simulink model "State_Flow_D"  (R2017a)
settings: Solver=FixedStepDiscrete  StartTime=0.0  StopTime=inf  FixedStep=0.001  RelTol=1e-3  EnableMultiTasking=on
libraries: xpcethercatlib x35, simulink x11, commutil2 x2
(part 3 of 3)

== matlab function State_Flow_D/Movimento/MATLAB Jin ==
  data: x input; y input; theta1 input; x_p output; theta2 input; theta1_p input; theta2_p input; y_p output
function [x_p, y_p] = fcn(x, y, theta1, theta2, theta1_p, theta2_p)

d = 0.09; 
l = 0.25;

N21 = -l*sin(theta1)*(x+d-l*cos(theta1)) + l*cos(theta1)*(y-l*sin(theta1));

N22 = -l*cos(theta2)*(y-l*sin(theta2))*(x+d-l*cos(theta1))/(x-d-l*cos(theta2)) + l*sin(theta2)*(x+d-l*cos(theta1));

D2 = y-l*sin(theta1) - (y-l*sin(theta2))*(x+d-l*cos(theta1))/(x-d-l*cos(theta2));

J21 = N21/D2;

J22 = N22/D2;

J11 = -(y-l*sin(theta2))/(x-d-l*cos(theta2))*(J21);

J12 = -(y-l*sin(theta2))/(x-d-l*cos(theta2))*(J22) -l*sin(theta2) + (y-l*sin(theta2))/(x-d-l*cos(theta2))*(l*cos(theta2));

x_p = J11*theta1_p + J12*theta2_p;
y_p = J21*theta1_p + J22*theta2_p;

== matlab function State_Flow_D/Movimento/Leggi di moto/Cerchio ==
  data: xc output; t input; yc output; T input; r input; xc_p output; yc_p output; xc_pp output; yc_pp output
function [xc, yc, xc_p, yc_p, xc_pp, yc_pp] = fcn(t, T, r)
xv = 0.4;
xj = 0.1;
x = t/T;
Ca = 1/((1-xv)*(xv-xj));
if ( x >= 0 && x < xj)            %acc crescente positiva
    f = Ca/xj*x;
    F = (1/2)*Ca/xj*x^2;
    G = (1/6)*Ca/xj*x^3;
    J = Ca/xj;

  elseif (x >= xj && x < (xv-xj))   %acc costante positiva
    f = Ca;
    F = Ca*x - (1/2)*Ca*xj;
    G = (1/2)*Ca*x^2 - (1/2)*Ca*xj*x + (1/6)*Ca*xj^2;
    J = 0;

  elseif( x>= (xv-xj) && x < xv)    %acc decrescente positiva
    f = -Ca/xj*x + Ca*xv/xj;
    F = -(1/2)*Ca/xj*x^2 + Ca/xj*xv*x - Ca*(xj + (1/2)/xj*xv^2 - xv);
    G = -(1/6)*Ca/xj*x^3 + (1/2)*Ca/xj*xv*x^2 - Ca*(xj + (1/2)/xj*xv^2 - xv)*x ...
        - (1/2)*Ca*xv^2  + (1/6)*Ca/xj*xv^3 + (1/2)*Ca*xv*xj;
    J = -Ca/xj;

  elseif( x>= xv && x < (1-xv))     %acc costante nulla
    f = 0;
    F = Ca*(xv - xj);
    G = Ca*(xv - xj)*x - (1/2)*Ca*xv^2 + (1/2)*Ca*xv*xj;
    J = 0;
    
  elseif( x>= (1-xv) && x < (1-xv+xj))   %acc decrescente negativa
    f = -Ca/xj*x + Ca/xj*(1-xv);
    F = -(1/2)*Ca/xj*x^2 + Ca/xj*(1-xv)*x + Ca*(xv-xj) - (1/2)*Ca/xj*(1-xv)^2;
    G = -(1/6)*Ca/xj*x^3 + (1/2)*Ca/xj*(1-xv)*x^2 + Ca*(xv-xj)*x - (1/2)*Ca/xj*(1-xv)^2*x ...
        - (1/2)*Ca*xv^2 + (1/2)*Ca*xv*xj + (1/6)*Ca/xj*(1-xv)^3;
    J = -Ca/xj;
    
  elseif( x>= (1-xv+xj) && x < (1-xj))   %acc costante negativa
    f = -Ca; 
    F = -Ca*x + Ca - (1/2)*Ca*xj;
    G = -(1/2)*Ca*x^2 + Ca*x - (1/2)*Ca*xj*x + 1 - Ca*(-(1/2)*xj + (1/6)*xj^2 + (1/2));
    J = 0;
    
  elseif( x>= (1-xj) && x <= 1)          %acc crescente negativa
    f = Ca/xj*(x-1);
    F = (1/2)*Ca/xj*x^2 - Ca/xj*x +(1/2)*Ca/xj;
    G = (1/6)*Ca/xj*x^3 - (1/2)*Ca/xj*x^2 +(1/2)*Ca/xj*x + 1 - (1/6)*Ca/xj;
    J = Ca/xj;
    
  else                                   %acc costante nulla
    f = 0;
    F = 0;
    G = 1;
    J = 0;
end
  
 alfa = G*2*pi;
 alfa_p = F*2*pi/T;
 alfa_pp = f*2*pi/(T^2);
 xc = r*cos(pi/2-alfa);
 yc = r*sin(pi/2-alfa) - r;
 xc_p = r*sin(pi/2-alfa)*alfa_p;
 yc_p = -r*cos(pi/2-alfa)*alfa_p;
 xc_pp = -r*cos(pi/2-alfa)*alfa_p^2 + r*sin(pi/2-alfa)*alfa_pp;
 yc_pp = -r*sin(pi/2-alfa)*alfa_p^2- r*cos(pi/2-alfa)*alfa_pp;

== matlab function State_Flow_D/Movimento/Leggi di moto/Quadrato ==
  data: xq output; yq output; t input; T input; h input; xq_p output; yq_p output; xq_pp output; yq_pp output
function [xq, yq, xq_p, yq_p, xq_pp, yq_pp] = fcn(t, T, h)
xv = 0.4;
xj = 0.1;
x1 = t/(0.5*T/4);
x2 = (t-0.5*T/4)/(T/4);
x3 = (t-1.5*T/4)/(T/4);
x4 = (t-2.5*T/4)/(T/4);
x5 = (t-3.5*T/4)/(0.5*T/4);
Ca = 1/((1-xv)*(xv-xj));
% Ca = 1/(xv*(1-xv));
% Cv = 1/(1-xv);


if t > 0 && t <= 0.5*T/4
  
  if ( x1 >= 0 && x1 < xj)            %acc crescente positiva
    f = Ca/xj*x1;
    F = (1/2)*Ca/xj*x1^2;
    G = (1/6)*Ca/xj*x1^3;
    J = Ca/xj;

  elseif (x1 >= xj && x1 < (xv-xj))   %acc costante positiva
    f = Ca;
    F = Ca*x1 - (1/2)*Ca*xj;
    G = (1/2)*Ca*x1^2 - (1/2)*Ca*xj*x1 + (1/6)*Ca*xj^2;
    J = 0;

  elseif( x1>= (xv-xj) && x1 < xv)    %acc decrescente positiva
    f = -Ca/xj*x1 + Ca*xv/xj;
    F = -(1/2)*Ca/xj*x1^2 + Ca/xj*xv*x1 - Ca*(xj + (1/2)/xj*xv^2 - xv);
    G = -(1/6)*Ca/xj*x1^3 + (1/2)*Ca/xj*xv*x1^2 - Ca*(xj + (1/2)/xj*xv^2 - xv)*x1 ...
        - (1/2)*Ca*xv^2  + (1/6)*Ca/xj*xv^3 + (1/2)*Ca*xv*xj;
    J = -Ca/xj;

  elseif( x1>= xv && x1 < (1-xv))     %acc costante nulla
    f = 0;
    F = Ca*(xv - xj);
    G = Ca*(xv - xj)*x1 - (1/2)*Ca*xv^2 + (1/2)*Ca*xv*xj;
    J = 0;
    
  elseif( x1>= (1-xv) && x1 < (1-xv+xj))   %acc decrescente negativa
    f = -Ca/xj*x1 + Ca/xj*(1-xv);
    F = -(1/2)*Ca/xj*x1^2 + Ca/xj*(1-xv)*x1 + Ca*(xv-xj) - (1/2)*Ca/xj*(1-xv)^2;
    G = -(1/6)*Ca/xj*x1^3 + (1/2)*Ca/xj*(1-xv)*x1^2 + Ca*(xv-xj)*x1 - (1/2)*Ca/xj*(1-xv)^2*x1 ...
        - (1/2)*Ca*xv^2 + (1/2)*Ca*xv*xj + (1/6)*Ca/xj*(1-xv)^3;
    J = -Ca/xj;
    
  elseif( x1>= (1-xv+xj) && x1 < (1-xj))   %acc costante negativa
    f = -Ca; 
    F = -Ca*x1 + Ca - (1/2)*Ca*xj;
    G = -(1/2)*Ca*x1^2 + Ca*x1 - (1/2)*Ca*xj*x1 + 1 - Ca*(-(1/2)*xj + (1/6)*xj^2 + (1/2));
    J = 0;
    
  elseif( x1>= (1-xj) && x1 <= 1)          %acc crescente negativa
    f = Ca/xj*(x1-1);
    F = (1/2)*Ca/xj*x1^2 - Ca/xj*x1 +(1/2)*Ca/xj;
    G = (1/6)*Ca/xj*x1^3 - (1/2)*Ca/xj*x1^2 +(1/2)*Ca/xj*x1 + 1 - (1/6)*Ca/xj;
    J = Ca/xj;
    
  else                                   %acc costante nulla
    f = 0;
    F = 0;
    G = 1;
    J = 0;
  end
    xq = G*h/2;
    xq_p = F*(h/2)/(T/4);
    yq = 0;
    yq_p = 0; 
    xq_pp = f*(h/2)/((T/4)^2);
    yq_pp = 0;

elseif t > 0.5*T/4 && t <= 1.5*T/4
    Ca = 1/((1-xv)*(xv-xj));
% Cj = Ca/xj;
  
  if ( x2 >= 0 && x2 < xj)            %acc crescente positiva
    f = Ca/xj*x2;
    F = (1/2)*Ca/xj*x2^2;
    G = (1/6)*Ca/xj*x2^3;
    J = Ca/xj;

  elseif (x2 >= xj && x2 < (xv-xj))   %acc costante positiva
    f = Ca;
    F = Ca*x2 - (1/2)*Ca*xj;
    G = (1/2)*Ca*x2^2 - (1/2)*Ca*xj*x2 + (1/6)*Ca*xj^2;
    J = 0;

  elseif( x2>= (xv-xj) && x2 < xv)    %acc decrescente positiva
    f = -Ca/xj*x2 + Ca*xv/xj;
    F = -(1/2)*Ca/xj*x2^2 + Ca/xj*xv*x2 - Ca*(xj + (1/2)/xj*xv^2 - xv);
    G = -(1/6)*Ca/xj*x2^3 + (1/2)*Ca/xj*xv*x2^2 - Ca*(xj + (1/2)/xj*xv^2 - xv)*x2 ...
        - (1/2)*Ca*xv^2  + (1/6)*Ca/xj*xv^3 + (1/2)*Ca*xv*xj;
    J = -Ca/xj;

  elseif( x2>= xv && x2 < (1-xv))     %acc costante nulla
    f = 0;
    F = Ca*(xv - xj);
    G = Ca*(xv - xj)*x2 - (1/2)*Ca*xv^2 + (1/2)*Ca*xv*xj;
    J = 0;
    
  elseif( x2>= (1-xv) && x2 < (1-xv+xj))   %acc decrescente negativa
    f = -Ca/xj*x2 + Ca/xj*(1-xv);
    F = -(1/2)*Ca/xj*x2^2 + Ca/xj*(1-xv)*x2 + Ca*(xv-xj) - (1/2)*Ca/xj*(1-xv)^2;
    G = -(1/6)*Ca/xj*x2^3 + (1/2)*Ca/xj*(1-xv)*x2^2 + Ca*(xv-xj)*x2 - (1/2)*Ca/xj*(1-xv)^2*x2 ...
        - (1/2)*Ca*xv^2 + (1/2)*Ca*xv*xj + (1/6)*Ca/xj*(1-xv)^3;
    J = -Ca/xj;
    
  elseif( x2>= (1-xv+xj) && x2 < (1-xj))   %acc costante negativa
    f = -Ca; 
    F = -Ca*x2 + Ca - (1/2)*Ca*xj;
    G = -(1/2)*Ca*x2^2 + Ca*x2 - (1/2)*Ca*xj*x2 + 1 - Ca*(-(1/2)*xj + (1/6)*xj^2 + (1/2));
    J = 0;
    
  elseif( x2>= (1-xj) && x2 <= 1)          %acc crescente negativa
    f = Ca/xj*(x2-1);
    F = (1/2)*Ca/xj*x2^2 - Ca/xj*x2 +(1/2)*Ca/xj;
    G = (1/6)*Ca/xj*x2^3 - (1/2)*Ca/xj*x2^2 +(1/2)*Ca/xj*x2 + 1 - (1/6)*Ca/xj;
    J = Ca/xj;
    
  else                                   %acc costante nulla
    f = 0;
    F = 0;
    G = 1;
    J = 0;
  end
    xq = h/2;
    xq_p = 0;
    yq = -G*h; 
    yq_p = -F*h/(T/4); 
    xq_pp = 0;
    yq_pp = -f*(h/2)/((T/4)^2);

elseif t > 1.5*T/4 && t <= 2.5*T/4
     Ca = 1/((1-xv)*(xv-xj));
% Cj = Ca/xj;
  
  if ( x3 >= 0 && x3 < xj)            %acc crescente positiva
    f = Ca/xj*x3;
    F = (1/2)*Ca/xj*x3^2;
    G = (1/6)*Ca/xj*x3^3;
    J = Ca/xj;

  elseif (x3 >= xj && x3 < (xv-xj))   %acc costante positiva
    f = Ca;
    F = Ca*x3 - (1/2)*Ca*xj;
    G = (1/2)*Ca*x3^2 - (1/2)*Ca*xj*x3 + (1/6)*Ca*xj^2;
    J = 0;

  elseif( x3>= (xv-xj) && x3 < xv)    %acc decrescente positiva
    f = -Ca/xj*x3 + Ca*xv/xj;
    F = -(1/2)*Ca/xj*x3^2 + Ca/xj*xv*x3 - Ca*(xj + (1/2)/xj*xv^2 - xv);
    G = -(1/6)*Ca/xj*x3^3 + (1/2)*Ca/xj*xv*x3^2 - Ca*(xj + (1/2)/xj*xv^2 - xv)*x3 ...
        - (1/2)*Ca*xv^2  + (1/6)*Ca/xj*xv^3 + (1/2)*Ca*xv*xj;
    J = -Ca/xj;

  elseif( x3>= xv && x3 < (1-xv))     %acc costante nulla
    f = 0;
    F = Ca*(xv - xj);
    G = Ca*(xv - xj)*x3 - (1/2)*Ca*xv^2 + (1/2)*Ca*xv*xj;
    J = 0;
    
  elseif( x3>= (1-xv) && x3 < (1-xv+xj))   %acc decrescente negativa
    f = -Ca/xj*x3 + Ca/xj*(1-xv);
    F = -(1/2)*Ca/xj*x3^2 + Ca/xj*(1-xv)*x3 + Ca*(xv-xj) - (1/2)*Ca/xj*(1-xv)^2;
    G = -(1/6)*Ca/xj*x3^3 + (1/2)*Ca/xj*(1-xv)*x3^2 + Ca*(xv-xj)*x3 - (1/2)*Ca/xj*(1-xv)^2*x3 ...
        - (1/2)*Ca*xv^2 + (1/2)*Ca*xv*xj + (1/6)*Ca/xj*(1-xv)^3;
    J = -Ca/xj;
    
  elseif( x3>= (1-xv+xj) && x3 < (1-xj))   %acc costante negativa
    f = -Ca; 
    F = -Ca*x3 + Ca - (1/2)*Ca*xj;
    G = -(1/2)*Ca*x3^2 + Ca*x3 - (1/2)*Ca*xj*x3 + 1 - Ca*(-(1/2)*xj + (1/6)*xj^2 + (1/2));
    J = 0;
    
  elseif( x3>= (1-xj) && x3 <= 1)          %acc crescente negativa
    f = Ca/xj*(x3-1);
    F = (1/2)*Ca/xj*x3^2 - Ca/xj*x3 +(1/2)*Ca/xj;
    G = (1/6)*Ca/xj*x3^3 - (1/2)*Ca/xj*x3^2 +(1/2)*Ca/xj*x3 + 1 - (1/6)*Ca/xj;
    J = Ca/xj;
    
  else                                   %acc costante nulla
    f = 0;
    F = 0;
    G = 1;
    J = 0;
  end
    xq = h/2-G*h;
    xq_p = -F*h/(T/4);
    yq = -h; 
    yq_p = 0; 
    xq_pp = -f*(h/2)/((T/4)^2);
    yq_pp = 0;
 
elseif t > 2.5*T/4 && t <= 3.5*T/4
   Ca = 1/((1-xv)*(xv-xj));
% Cj = Ca/xj;
  
  if ( x4 >= 0 && x4 < xj)            %acc crescente positiva
    f = Ca/xj*x4;
    F = (1/2)*Ca/xj*x4^2;
    G = (1/6)*Ca/xj*x4^3;
    J = Ca/xj;

  elseif (x4 >= xj && x4 < (xv-xj))   %acc costante positiva
    f = Ca;
    F = Ca*x4 - (1/2)*Ca*xj;
    G = (1/2)*Ca*x4^2 - (1/2)*Ca*xj*x4 + (1/6)*Ca*xj^2;
    J = 0;

  elseif( x4>= (xv-xj) && x4 < xv)    %acc decrescente positiva
    f = -Ca/xj*x4 + Ca*xv/xj;
    F = -(1/2)*Ca/xj*x4^2 + Ca/xj*xv*x4 - Ca*(xj + (1/2)/xj*xv^2 - xv);
    G = -(1/6)*Ca/xj*x4^3 + (1/2)*Ca/xj*xv*x4^2 - Ca*(xj + (1/2)/xj*xv^2 - xv)*x4 ...
        - (1/2)*Ca*xv^2  + (1/6)*Ca/xj*xv^3 + (1/2)*Ca*xv*xj;
    J = -Ca/xj;

  elseif( x4>= xv && x4 < (1-xv))     %acc costante nulla
    f = 0;
    F = Ca*(xv - xj);
    G = Ca*(xv - xj)*x4 - (1/2)*Ca*xv^2 + (1/2)*Ca*xv*xj;
    J = 0;
    
  elseif( x4>= (1-xv) && x4 < (1-xv+xj))   %acc decrescente negativa
    f = -Ca/xj*x4 + Ca/xj*(1-xv);
    F = -(1/2)*Ca/xj*x4^2 + Ca/xj*(1-xv)*x4 + Ca*(xv-xj) - (1/2)*Ca/xj*(1-xv)^2;
    G = -(1/6)*Ca/xj*x4^3 + (1/2)*Ca/xj*(1-xv)*x4^2 + Ca*(xv-xj)*x4 - (1/2)*Ca/xj*(1-xv)^2*x4 ...
        - (1/2)*Ca*xv^2 + (1/2)*Ca*xv*xj + (1/6)*Ca/xj*(1-xv)^3;
    J = -Ca/xj;
    
  elseif( x4>= (1-xv+xj) && x4 < (1-xj))   %acc costante negativa
    f = -Ca; 
    F = -Ca*x4 + Ca - (1/2)*Ca*xj;
    G = -(1/2)*Ca*x4^2 + Ca*x4 - (1/2)*Ca*xj*x4 + 1 - Ca*(-(1/2)*xj + (1/6)*xj^2 + (1/2));
    J = 0;
    
  elseif( x4>= (1-xj) && x4 <= 1)          %acc crescente negativa
    f = Ca/xj*(x4-1);
    F = (1/2)*Ca/xj*x4^2 - Ca/xj*x4 +(1/2)*Ca/xj;
    G = (1/6)*Ca/xj*x4^3 - (1/2)*Ca/xj*x4^2 +(1/2)*Ca/xj*x4 + 1 - (1/6)*Ca/xj;
    J = Ca/xj;
    
  else                                   %acc costante nulla
    f = 0;
    F = 0;
    G = 1;
    J = 0;
  end
    xq = -h/2;
    xq_p = 0;
    yq = -h + G*h;
    yq_p = F*h/(T/4); 
    xq_pp = 0;
    yq_pp = f*(h/2)/((T/4)^2);

elseif t > 3.5*T/4 && t <= 4*T/4
   Ca = 1/((1-xv)*(xv-xj));
% Cj = Ca/xj;
  
  if ( x5 >= 0 && x5 < xj)            %acc crescente positiva
    f = Ca/xj*x5;
    F = (1/2)*Ca/xj*x5^2;
    G = (1/6)*Ca/xj*x5^3;
    J = Ca/xj;

  elseif (x5 >= xj && x5 < (xv-xj))   %acc costante positiva
    f = Ca;
    F = Ca*x5 - (1/2)*Ca*xj;
    G = (1/2)*Ca*x5^2 - (1/2)*Ca*xj*x5 + (1/6)*Ca*xj^2;
    J = 0;

  elseif( x5>= (xv-xj) && x5 < xv)    %acc decrescente positiva
    f = -Ca/xj*x5 + Ca*xv/xj;
    F = -(1/2)*Ca/xj*x5^2 + Ca/xj*xv*x5 - Ca*(xj + (1/2)/xj*xv^2 - xv);
    G = -(1/6)*Ca/xj*x5^3 + (1/2)*Ca/xj*xv*x5^2 - Ca*(xj + (1/2)/xj*xv^2 - xv)*x5 ...
        - (1/2)*Ca*xv^2  + (1/6)*Ca/xj*xv^3 + (1/2)*Ca*xv*xj;
    J = -Ca/xj;

  elseif( x5>= xv && x5 < (1-xv))     %acc costante nulla
    f = 0;
    F = Ca*(xv - xj);
    G = Ca*(xv - xj)*x5 - (1/2)*Ca*xv^2 + (1/2)*Ca*xv*xj;
    J = 0;
    
  elseif( x5>= (1-xv) && x5 < (1-xv+xj))   %acc decrescente negativa
    f = -Ca/xj*x5 + Ca/xj*(1-xv);
    F = -(1/2)*Ca/xj*x5^2 + Ca/xj*(1-xv)*x5 + Ca*(xv-xj) - (1/2)*Ca/xj*(1-xv)^2;
    G = -(1/6)*Ca/xj*x5^3 + (1/2)*Ca/xj*(1-xv)*x5^2 + Ca*(xv-xj)*x5 - (1/2)*Ca/xj*(1-xv)^2*x5 ...
        - (1/2)*Ca*xv^2 + (1/2)*Ca*xv*xj + (1/6)*Ca/xj*(1-xv)^3;
    J = -Ca/xj;
    
  elseif( x5>= (1-xv+xj) && x5 < (1-xj))   %acc costante negativa
    f = -Ca; 
    F = -Ca*x5 + Ca - (1/2)*Ca*xj;
    G = -(1/2)*Ca*x5^2 + Ca*x5 - (1/2)*Ca*xj*x5 + 1 - Ca*(-(1/2)*xj + (1/6)*xj^2 + (1/2));
    J = 0;
    
  elseif( x5>= (1-xj) && x5 <= 1)          %acc crescente negativa
    f = Ca/xj*(x5-1);
    F = (1/2)*Ca/xj*x5^2 - Ca/xj*x5 +(1/2)*Ca/xj;
    G = (1/6)*Ca/xj*x5^3 - (1/2)*Ca/xj*x5^2 +(1/2)*Ca/xj*x5 + 1 - (1/6)*Ca/xj;
    J = Ca/xj;
    
  else                                   %acc costante nulla
    f = 0;
    F = 0;
    G = 1;
    J = 0;
  end
    xq = -h/2 + G*h/2;
    xq_p = F*h/2/(T/4);
    yq = 0
    yq_p = 0; 
    xq_pp = f*(h/2)/((T/4)^2);
    yq_pp = 0;
else
xq = 0;
yq = 0;
xq_p = 0;
yq_p = 0; 
xq_pp = 0;
yq_pp = 0;
end

== matlab function State_Flow_D/Movimento/Leggi di moto/g ==
  data: x output; y output; x_p output; t input; l input; T input; y_p output; x_pp output; y_pp output
function [x, y, x_p,y_p, x_pp, y_pp] = fcn(t, l, T)
 Tt = T/32;
 t1 = (t-0*Tt/2)/(Tt/2);
 t2 = (t-1*Tt/2)/Tt;
 t3 = (t-3*Tt/2)/(Tt/2);
 t4 = (t-4*Tt/2)/(Tt/2);
 t5 = (t-5*Tt/2)/Tt;
 t6 = (t-7*Tt/2)/Tt;
 t7 = (t-9*Tt/2)/Tt;
 t8 = (t-11*Tt/2)/(Tt/2);
 t9 = (t-12*Tt/2)/(Tt/2);
 t10 = (t-13*Tt/2)/Tt;
 t11 = (t-15*Tt/2)/(Tt/2);
 t12 = (t-16*Tt/2)/(Tt/2);
 t13 = (t-17*Tt/2)/Tt;
 t14 = (t-19*Tt/2)/(Tt/2);
 t15 = (t-20*Tt/2)/(Tt/2);
 t16 = (t-21*Tt/2)/Tt;
 t17 = (t-23*Tt/2)/Tt;
 t18 = (t-25*Tt/2)/Tt;
 t19 = (t-27*Tt/2)/(Tt/2);
 t20 = (t-28*Tt/2)/(Tt/2);
 t21 = (t-29*Tt/2)/Tt;
 t22 = (t-31*Tt/2)/(Tt/2);
 t23 = (t-32*Tt/2)/(Tt/2);
 t24 = (t-33*Tt/2)/Tt;
 t25 = (t-35*Tt/2)/(Tt/2);
 t26 = (t-36*Tt/2)/(Tt/2);
 t27 = (t-37*Tt/2)/Tt;
 t28 = (t-39*Tt/2)/Tt;
 t29 = (t-41*Tt/2)/Tt;
 t30 = (t-43*Tt/2)/(Tt/2);
 t31 = (t-44*Tt/2)/(Tt/2);
 t32 = (t-45*Tt/2)/Tt;
 t33 = (t-47*Tt/2)/(Tt/2);
 t34 = (t-48*Tt/2)/(Tt/2);
 t35 = (t-49*Tt/2)/Tt;
 t36 = (t-51*Tt/2)/(Tt/2);
 t37 = (t-52*Tt/2)/(Tt/2);
 t38 = (t-53*Tt/2)/Tt;
 t39 = (t-55*Tt/2)/Tt;
 t40 = (t-57*Tt/2)/Tt;
 t41 = (t-59*Tt/2)/(Tt/2);
 t42 = (t-60*Tt/2)/(Tt/2);
 t43 = (t-61*Tt/2)/Tt;
 t44 = (t-63*Tt/2)/(Tt/2);
 
 if t > 0 && t <= Tt/2 % 1
     [G, F, f] = ldm7t(t1);
     x = 0;
     x_p = 0;
     y = -G*l;
     y_p = -F*l/(Tt/2);
     x_pp = 0;
     y_pp = -f*l/((Tt/2)^2);
     
 elseif t > Tt/2 && t <= 3*Tt/2 % 2
     [G, F, f] = ldm7t(t2);
     x = G*3*l;
     x_p = F*3*l/Tt;
     y = -l;
     y_p = 0;
     x_pp = f*l/((Tt)^2);
     y_pp = 0;
     
 elseif t > 3*Tt/2 && t <= 4*Tt/2 % 3
     [G, F, f] = ldm7t(t3);
     x = 3*l;
     x_p = 0;
     y = -l + G*l;
     y_p = F*l/(Tt/2);
     x_pp = 0;
     y_pp = f*l/((Tt/2)^2);
     
  elseif t > 4*Tt/2 && t <= 5*Tt/2 % 4
     [G, F, f] = ldm7t(t4);
     x = 3*l - G*l;
     x_p = -F*l/(Tt/2);
     y = 0;
     y_p = 0;
     x_pp = -f*l/((Tt/2)^2);
     y_pp = 0;
     
  elseif t > 5*Tt/2 && t <= 7*Tt/2 % 5
     [G, F, f] = ldm7t(t5);
     x = 2*l;
     x_p = 0;
     y = -G*3*l;
     y_p = -F*3*l/Tt;
     x_pp = 0;
     y_pp = -f*l/((Tt)^2);
     
  elseif t > 7*Tt/2 && t <= 9*Tt/2 % 6
     [G, F, f] = ldm7t(t6);
     x = 2*l + G*3*l;
     x_p = F*3*l/Tt;
     y = -3*l;
     y_p = 0;
     x_pp = f*l/((Tt)^2);
     y_pp = 0;
     
  elseif t > 9*Tt/2 && t <= 11*Tt/2 % 7
     [G, F, f] = ldm7t(t7);
     x = 5*l;
     x_p = 0;
     y = -3*l + G*3*l;
     y_p = -F*3*l/Tt;
     x_pp = 0;
     y_pp = f*l/((Tt)^2);
     
   elseif t > 11*Tt/2 && t <= 12*Tt/2 % 8
     [G, F, f] = ldm7t(t8);
     x = 5*l - G*l;
     x_p = -F*l/(Tt/2);
     y = 0;
     y_p = 0;  
     x_pp = -f*l/((Tt/2)^2);
     y_pp = 0;
     
   elseif t > 12*Tt/2 && t <= 13*Tt/2 % 9
     [G, F, f] = ldm7t(t9);
     x = 4*l;
     x_p = 0;
     y = -G*l;
     y_p = -F*l/(Tt/2);  
     x_pp = 0;
     y_pp = -f*l/((Tt/2)^2);
     
   elseif t > 13*Tt/2 && t <= 15*Tt/2 % 10
     [G, F, f] = ldm7t(t10);
     x = 4*l + G*3*l;
     x_p = F*3*l/Tt;
     y = -l;
     y_p = 0;
     x_pp = f*l/((Tt)^2);
     y_pp = 0;
     
   elseif t > 15*Tt/2 && t <= 16*Tt/2 % 11
     [G, F, f] = ldm7t(t11);
     x = 7*l;
     x_p = 0;
     y = -l + G*l;
     y_p = F*l/(Tt/2);
     x_pp = 0;
     y_pp = f*l/((Tt/2)^2);
     
   elseif t > 16*Tt/2 && t <= 17*Tt/2 % 12
     [G, F, f] = ldm7t(t12);
     x = 7*l - G*l;
     x_p = -F*l/(Tt/2);
     y = 0;
     y_p = 0;
     x_pp = -f*l/((Tt/2)^2);
     y_pp = 0;
     
   elseif t > 17*Tt/2 && t <= 19*Tt/2 % 13
     [G, F, f] = ldm7t(t13);
     x = 6*l;
     x_p = 0;
     y = -G*3*l;
     y_p = -F*3*l/Tt;
     x_pp = 0;
     y_pp = -f*l/((Tt)^2);
     
   elseif t > 19*Tt/2 && t <= 20*Tt/2 % 14
     [G, F, f] = ldm7t(t14);
     x = 6*l + G*l;
     x_p = F*l/(Tt/2);
     y = -3*l;
     y_p = 0;
     x_pp = f*l/((Tt/2)^2);
     y_pp = 0;
     
   elseif t > 20*Tt/2 && t <= 21*Tt/2 % 15
     [G, F, f] = ldm7t(t15);
     x = 7*l;
     x_p = 0;
     y = -3*l + G*l;
     y_p = F*l/(Tt/2);
     x_pp = 0;
     y_pp = f*l/((Tt/2)^2);
     
   elseif t > 21*Tt/2 && t <= 23*Tt/2 % 16
     [G, F, f] = ldm7t(t16);
     x = 7*l - G*3*l;
     x_p = -F*3*l/Tt;
     y = -2*l;
     y_p = 0;
     x_pp = -f*l/((Tt)^2);
     y_pp = 0;
     
   elseif t > 23*Tt/2 && t <= 25*Tt/2 % 17
     [G, F, f] = ldm7t(t17);
     x = 4*l;
     x_p = 0;
     y = -2*l - 3*G*l;
     y_p = -F*3*l/Tt;
     x_pp = 0;
     y_pp = -f*l/((Tt)^2);
     
   elseif t > 25*Tt/2 && t <= 27*Tt/2 % 18
     [G, F, f] = ldm7t(t18);
     x = 4*l + 3*G*l;
     x_p = F*3*l/Tt;
     y = -5*l;
     y_p = 0;
     x_pp = f*l/((Tt)^2);
     y_pp = 0;
     
   elseif t > 27*Tt/2 && t <= 28*Tt/2 % 19
     [G, F, f] = ldm7t(t19);
     x = 7*l;
     x_p = 0;
     y = -5*l + G*l;
     y_p = F*l/(Tt/2);
     x_pp = 0;
     y_pp = f*l/((Tt/2)^2);
     
   elseif t > 28*Tt/2 && t <= 29*Tt/2 % 20
     [G, F, f] = ldm7t(t20);
     x = 7*l - G*l;
     x_p = -F*l/(Tt/2);
     y = -4*l;
     y_p = 0;
     x_pp = -f*l/((Tt/2)^2);
     y_pp = 0;
     
   elseif t > 29*Tt/2 && t <= 31*Tt/2 % 21
     [G, F, f] = ldm7t(t21);
     x = 6*l;
     x_p = 0;
     y = -4*l - 3*G*l;
     y_p = -F*3*l/Tt;
     x_pp = 0;
     y_pp = -f*l/((Tt)^2);
     
   elseif t > 31*Tt/2 && t <= 32*Tt/2 % 22
     [G, F, f] = ldm7t(t22);
     x = 6*l + G*l;
     x_p = F*l/(Tt/2);
     y = -7*l;
     y_p = 0;
     x_pp = f*l/((Tt/2)^2);
     y_pp = 0;
     
   elseif t > 32*Tt/2 && t <= 33*Tt/2 % 23
     [G, F, f] = ldm7t(t23);
     x = 7*l;
     x_p = 0;
     y = -7*l + G*l;
     y_p = F*l/(Tt/2);
     x_pp = 0;
     y_pp = f*l/((Tt/2)^2);
     
   elseif t > 33*Tt/2 && t <= 35*Tt/2 % 24
     [G, F, f] = ldm7t(t24);
     x = 7*l - 3*G*l;
     x_p = -F*3*l/Tt;
     y = -6*l;
     y_p = 0;
     x_pp = -f*l/((Tt)^2);
     y_pp = 0;
     
   elseif t > 35*Tt/2 && t <= 36*Tt/2 % 25
     [G, F, f] = ldm7t(t25);
     x = 4*l;
     x_p = 0;
     y = -6*l - G*l;
     y_p = -F*l/(Tt/2);
     x_pp = 0;
     y_pp = -f*l/((Tt/2)^2);
     
   elseif t > 36*Tt/2 && t <= 37*Tt/2 % 26
     [G, F, f] = ldm7t(t26);
     x = 4*l + G*l;
     x_p = F*l/(Tt/2);
     y = -7*l;
     y_p = 0;
     x_pp = f*l/((Tt/2)^2);
     y_pp = 0;
     
   elseif t > 37*Tt/2 && t <= 39*Tt/2 % 27
     [G, F, f] = ldm7t(t27);
     x = 5*l;
     x_p = 0;
     y = -7*l + 3*G*l;
     y_p = F*3*l/Tt;
     x_pp = 0;
     y_pp = f*l/((Tt)^2);
     
   elseif t > 39*Tt/2 && t <= 41*Tt/2 % 28
     [G, F, f] = ldm7t(t28);
     x = 5*l - 3*G*l;
     x_p = -F*3*l/Tt;
     y = -4*l;
     y_p = 0;
     x_pp = f*l/((Tt)^2);
     y_pp = 0;
     
   elseif t > 41*Tt/2 && t <= 43*Tt/2 % 29
     [G, F, f] = ldm7t(t29);
     x = 2*l;
     x_p = 0;
     y = -4*l - G*3*l;
     y_p = -F*3*l/Tt;
     x_pp = 0;
     y_pp = -f*l/((Tt)^2);
     
   elseif t > 43*Tt/2 && t <= 44*Tt/2 % 30
     [G, F, f] = ldm7t(t30);
     x = 2*l + G*l;
     x_p = F*l/(Tt/2);
     y = -7*l;
     y_p = 0;
     x_pp = f*l/((Tt/2)^2);
     y_pp = 0;
     
   elseif t > 44*Tt/2 && t <= 45*Tt/2 % 31
     [G, F, f] = ldm7t(t31);
     x = 3*l;
     x_p = 0;
     y = -7*l + G*l;
     y_p = F*l/(Tt/2);
     x_pp = 0;
     y_pp = f*l/((Tt/2)^2);
     
   elseif t > 45*Tt/2 && t <= 47*Tt/2 % 32
     [G, F, f] = ldm7t(t32);
     x = 3*l - 3*G*l;
     x_p = -F*3*l/Tt;
     y = -6*l;
     y_p = 0;
     x_pp = -f*l/((Tt)^2);
     y_pp = 0;
     
   elseif t > 47*Tt/2 && t <= 48*Tt/2 % 33
     [G, F, f] = ldm7t(t33);
     x = 0;
     x_p = 0;
     y = -6*l - G*l;
     y_p = -F*l/(Tt/2);
     x_pp = 0;
     y_pp = -f*l/((Tt/2)^2);
     
   elseif t > 48*Tt/2 && t <= 49*Tt/2 % 34
     [G, F, f] = ldm7t(t34);
     x = G*l;
     x_p = F*l/(Tt/2);
     y = -7*l;
     y_p = 0;
     x_pp = f*l/((Tt/2)^2);
     y_pp = 0;
     
   elseif t > 49*Tt/2 && t <= 51*Tt/2 % 35
     [G, F, f] = ldm7t(t35);
     x = l;
     x_p = 0;
     y = -7*l + 3*G*l;
     y_p = F*3*l/Tt;
     x_pp = 0;
     y_pp = f*l/((Tt)^2);
     
   elseif t > 51*Tt/2 && t <= 52*Tt/2 % 36
     [G, F, f] = ldm7t(t36);
     x = l - G*l;
     x_p = -F*l/(Tt/2);
     y = -4*l;
     y_p = 0;
     x_pp = -f*l/((Tt/2)^2);
     y_pp = 0;
     
   elseif t > 52*Tt/2 && t <= 53*Tt/2 % 37
     [G, F, f] = ldm7t(t37);
     x = 0;
     x_p = 0;
     y = -4*l - G*l;
     y_p = -F*l/(Tt/2);
     x_pp = 0;
     y_pp = -f*l/((Tt/2)^2);
     
   elseif t > 53*Tt/2 && t <= 55*Tt/2 % 38
     [G, F, f] = ldm7t(t38);
     x = 3*G*l;
     x_p = F*3*l/Tt;
     y = -5*l;
     y_p = 0;
     x_pp = f*l/((Tt)^2);
     y_pp = 0;
     
   elseif t > 55*Tt/2 && t <= 57*Tt/2 % 39
     [G, F, f] = ldm7t(t39);
     x = 3*l;
     x_p = 0;
     y = -5*l + G*3*l;
     y_p = F*3*l/Tt;
     x_pp = 0;
     y_pp = f*l/((Tt)^2);
     
   elseif t > 57*Tt/2 && t <= 59*Tt/2 % 40
     [G, F, f] = ldm7t(t40);
     x = 3*l -G*3*l;
     x_p = -F*3*l/Tt;
     y = -2*l;
     y_p = 0;
     x_pp = -f*l/((Tt)^2);
     y_pp = 0;
     
   elseif t > 59*Tt/2 && t <= 60*Tt/2 % 41
     [G, F, f] = ldm7t(t41);
     x = 0;
     x_p = 0;
     y = -2*l - G*l;
     y_p = -F*l/(Tt/2);
     x_pp = 0;
     y_pp = -f*l/((Tt/2)^2);
     
   elseif t > 60*Tt/2 && t <= 61*Tt/2 % 42
     [G, F, f] = ldm7t(t42);
     x = G*l;
     x_p = F*l/(Tt/2);
     y = -3*l;
     y_p = 0;
     x_pp = f*l/((Tt/2)^2);
     y_pp = 0;
     
   elseif t > 61*Tt/2 && t <= 63*Tt/2 % 43
     [G, F, f] = ldm7t(t43);
     x = l;
     x_p = 0;
     y = -3*l + 3*G*l;
     y_p = F*3*l/Tt;
     x_pp = 0;
     y_pp = f*l/((Tt)^2);
     
   elseif t > 63*Tt/2 && t <= 64*Tt/2 % 44
     [G, F, f] = ldm7t(t44);
     x = l - G*l;
     x_p = -F*l/(Tt/2);
     y = 0;
     y_p = 0;
     x_pp = -f*l/((Tt/2)^2);
     y_pp = 0;
     
 else
     x = 0;
     x_p = 0;
     y = 0;
     y_p = 0;
     x_pp = 0;
     y_pp = 0;
 end

== matlab function State_Flow_D/Movimento/Velocita vite /Vel Asse A conv ==
  data: vA input; vel_A_conv output
function vel_A_conv = fcn(vA)
vel_A_conv = (vA)  *(2*pi)/163840/64;

== matlab function State_Flow_D/Movimento/Leggi di moto/spirale ==
  data: xs output; t input; ys output; T input; xs_p output; ys_p output; Rmax input; N input; Rmin input; T1 input; xs_pp output; ys_pp output
function [xs, ys, xs_p, ys_p, xs_pp, ys_pp] = fcn(t, T, Rmax, N, Rmin, T1)

t1 = t/T1;
t2 = (t-T1)/T;
if t >= 0 && t <= T1
    [G, F, f] = ldm7t(t1);
     xs = G*Rmin;
     xs_p = F*Rmin/T1;
     xs_pp = f*Rmin/(T1^2);
     ys = 0;
     ys_p = 0;
     ys_pp = 0;
elseif t > T1 && t <= T1+T 
    [G, F, f] = ldm7t(t2);
    r = Rmin + G*Rmax;
    r_p = F*Rmax/T;
    r_pp = f*Rmax/(T^2);
    alfa = G*N*2*pi;
    alfa_p = F*N*2*pi/T;
    alfa_pp = f*N*2*pi/(T^2);
    xs = r*cos(alfa);
    ys = r*sin(alfa);
    xs_p = -r*sin(alfa)*alfa_p + r_p*cos(alfa);
    ys_p = r*cos(alfa)*alfa_p + r_p*sin(alfa);
    xs_pp = -r_p*sin(alfa)*alfa_p - r*(cos(alfa)*alfa_p^2 + sin(alfa)*alfa_pp) + r_pp*cos(alfa) - r_p*sin(alfa)*alfa_p;
    ys_pp = r_p*cos(alfa)*alfa_p + r*(-sin(alfa)*alfa_p^2 + cos(alfa)*alfa_pp) + r_pp*sin(alfa) + r_p*cos(alfa)*alfa_p;
else
     xs = (Rmin+Rmax)*cos(N*2*pi);
     xs_p = 0;
     ys = (Rmin+Rmax)*sin(N*2*pi);
     ys_p = 0;
     xs_pp =0;
     ys_pp =0;
 end

== matlab function State_Flow_D/Movimento/Cinematica Inversa Acc ==
  data: x input; y input; x_p input; y_p input; x_pp input; y_pp input; theta1 input; theta2 input; theta1_pp output; theta1_p input; theta2_p input; theta2_pp output
function [theta1_pp, theta2_pp] = CinInvAcc(x, y, x_p, y_p, x_pp, y_pp, theta1, theta2, theta1_p,theta2_p)

d = 0.09; 
l = 0.25;

N21 = -l*sin(theta1)*(x+d-l*cos(theta1)) + l*cos(theta1)*(y-l*sin(theta1));

N22 = -l*cos(theta2)*(y-l*sin(theta2))*(x+d-l*cos(theta1))/(x-d-l*cos(theta2)) + l*sin(theta2)*(x+d-l*cos(theta1));

D2 = y-l*sin(theta1) - (y-l*sin(theta2))*(x+d-l*cos(theta1))/(x-d-l*cos(theta2));

J21 = N21/D2;

J22 = N22/D2;

J11 = -(y-l*sin(theta2))/(x-d-l*cos(theta2))*(J21);

J12 = -(y-l*sin(theta2))/(x-d-l*cos(theta2))*(J22) -l*sin(theta2) + (y-l*sin(theta2))/(x-d-l*cos(theta2))*(l*cos(theta2));

J = [J11 J12; J21 J22];

N11 = -(2*l*x*sin(theta1) - 2*l*y*cos(theta1) + 2*d*l*sin(theta1))*(2*x-2*d-2*d*cos(theta2))*(2*y-2*l*sin(theta2));

N12 = ((2*l*x*sin(theta2) - 2*l*y*cos(theta2) - 2*d*l*sin(theta2))*(2*x +2*d -2*l*cos(theta1))*(2*y - 2*l*sin(theta2)) - (2*l*x*sin(theta2) -...
    2*l*y*cos(theta2) - 2*d*l*sin(theta2))*(2*y - 2*l*sin(theta2))*(2*x + 2*d - 2*l*cos(theta1)) +...
    (2*y -  2*l*sin(theta1))*(2*x +2*d - 2*l*cos(theta2)));


D1 = (2*x -2*d -2*l*cos(theta2))*(2*y -2*l*sin(theta2))*(2*x +2*d -2*l*cos(theta1)) + (2*y -2*l*sin(theta1))*(2*x +2*d -2*l*cos(theta2));

D2 = (2*y -2*l*sin(theta2))*(2*x +2*d -2*l*cos(theta1)) + (2*y -2*l*sin(theta1))*(2*x +2*d -2*l*cos(theta2));


N21 = (2*l*x*sin(theta1) - 2*l*y*cos(theta1) + 2*d*l*sin(theta1))*(2*x -2*d -2*d*cos(theta2));


N22 = -(2*l*x*sin(theta2) - 2*l*y*cos(theta2) - 2*d*l*sin(theta2))*(2*x +2*d -2*l*cos(theta1));
    
N11_p = (sin(theta2)/2 - 2*y)*((9*sin(theta2)*theta2_p)/50 + 2*x_p)*((9*sin(theta1))/200 - (cos(theta1)*y)/2 + (sin(theta1)*x)/2) -...
    ((cos(theta2)*theta2_p)/2 - 2*y_p)*((9*cos(theta2))/50 - 2*x + 9/50)*((9*sin(theta1))/200 - (cos(theta1)*y)/2 + (sin(theta1)*x)/2) -...
    (sin(theta2)/2 - 2*y)*((9*cos(theta2))/50 - 2*x + 9/50)*((9*cos(theta1)*theta1_p)/200 - (cos(theta1)*y_p)/2 + (sin(theta1)*x_p)/2 +...
    (cos(theta1)*x*theta1_p)/2 + (sin(theta1)*y*theta1_p)/2);

N12_p= - ((cos(theta1)*theta1_p)/2 - 2*y_p)*(2*x - cos(theta2)/2 + 9/50) - (sin(theta1)/2 - 2*y)*((sin(theta2)*theta2_p)/2 + 2*x_p);
 
N21_p = ((9*sin(theta2)*theta2_p)/50 + 2*x_p)*((9*sin(theta1))/200 - (cos(theta1)*y)/2 + (sin(theta1)*x)/2) - ((9*cos(theta2))/50 -...
2*x + 9/50)*((9*cos(theta1)*theta1_p)/200 - (cos(theta1)*y_p)/2 + (sin(theta1)*x_p)/2 +(cos(theta1)*x*theta1_p)/2 + (sin(theta1)*y*theta1_p)/2);

N22_p = ((sin(theta1)*theta1_p)/2 + 2*x_p)*((9*sin(theta2))/200 + (cos(theta2)*y)/2 - (sin(theta2)*x)/2) - (2*x - cos(theta1)/2 + 9/50)*...
    ((sin(theta2)*x_p)/2 - (cos(theta2)*y_p)/2 - (9*cos(theta2)*theta2_p)/200 + (cos(theta2)*x*theta2_p)/2 + (sin(theta2)*y*theta2_p)/2);

D1_p = (sin(theta2)/2 - 2*y)*((sin(theta1)*theta1_p)/2 + 2*x_p)*(cos(theta2)/2 - 2*x + 9/50) - (sin(theta1)/2 - 2*y)*((sin(theta2)*theta2_p)/2 +...
    2*x_p) - ((cos(theta1)*theta1_p)/2 - 2*y_p)*(2*x - cos(theta2)/2 + 9/50) - (sin(theta2)/2 - 2*y)*((sin(theta2)*theta2_p)/2 + 2*x_p)*...
    (2*x - cos(theta1)/2 + 9/50) + ((cos(theta2)*theta1_p)/2 - 2*y_p)*(2*x - cos(theta1)/2 + 9/50)*(cos(theta2)/2 - 2*x + 9/50);

D2_p = - ((cos(theta1)*theta1_p)/2 - 2*y_p)*(2*x - cos(theta2)/2 + 9/50) - ((cos(theta2)*theta2_p)/2 - 2*y_p)*(2*x - cos(theta1)/2 + 9/50) -...
    (sin(theta2)/2 - 2*y)*((sin(theta1)*theta1_p)/2 + 2*x_p) - (sin(theta1)/2 - 2*y)*((sin(theta2)*theta2_p)/2 + 2*x_p);

J_p11 = ((l*cos(theta1)*(y - l*sin(theta1)) - l*sin(theta1)*(d + x - l*cos(theta1)))*(y_p - l*cos(theta2)*theta2_p))/((d - x + l*cos(theta2))*(y - l*sin(theta1) + ((y - l*sin(theta2))*(d + x - l*cos(theta1)))/(d - x + l*cos(theta2)))) - ((y - l*sin(theta2))*(l*sin(theta1)*(x_p + l*sin(theta1)*theta1_p) - l*cos(theta1)*(y_p - l*cos(theta1)*theta1_p) + l*sin(theta1)*(y - l*sin(theta1))*theta1_p + l*cos(theta1)*theta1_p*(d + x - l*cos(theta1))))/((d - x + l*cos(theta2))*(y - l*sin(theta1) + ((y - l*sin(theta2))*(d + x - l*cos(theta1)))/(d - x + l*cos(theta2)))) + ((x_p + l*sin(theta2)*theta2_p)*(y - l*sin(theta2))*(l*cos(theta1)*(y - l*sin(theta1)) - l*sin(theta1)*(d + x - l*cos(theta1))))/((d - x + l*cos(theta2))^2*(y - l*sin(theta1) + ((y - l*sin(theta2))*(d + x - l*cos(theta1)))/(d - x + l*cos(theta2)))) - ((y - l*sin(theta2))*(l*cos(theta1)*(y - l*sin(theta1)) - l*sin(theta1)*(d + x - l*cos(theta1)))*(y_p + ((x_p + l*sin(theta1)*theta1_p)*(y - l*sin(theta2)))/(d - x + l*cos(theta2)) + ((y_p - l*cos(theta2)*theta2_p)*(d + x - l*cos(theta1)))/(d - x + l*cos(theta2)) - l*cos(theta1)*theta1_p + ((x_p + l*sin(theta2)*theta2_p)*(y - l*sin(theta2))*(d + x - l*cos(theta1)))/(d - x + l*cos(theta2))^2))/((d - x + l*cos(theta2))*(y - l*sin(theta1) + ((y - l*sin(theta2))*(d + x - l*cos(theta1)))/(d - x + l*cos(theta2)))^2);
 
 
J_p12 = ((y - l*sin(theta2))*(l*sin(theta2)*(x_p + l*sin(theta1)*theta1_p) + l*cos(theta2)*theta2_p*(d + x - l*cos(theta1)) + (l*cos(theta2)*(x_p + l*sin(theta1)*theta1_p)*(y - l*sin(theta2)))/(d - x + l*cos(theta2)) + (l*cos(theta2)*(y_p - l*cos(theta2)*theta2_p)*(d + x - l*cos(theta1)))/(d - x + l*cos(theta2)) - (l*sin(theta2)*(y - l*sin(theta2))*theta2_p*(d + x - l*cos(theta1)))/(d - x + l*cos(theta2)) + (l*cos(theta2)*(x_p + l*sin(theta2)*theta2_p)*(y - l*sin(theta2))*(d + x - l*cos(theta1)))/(d - x + l*cos(theta2))^2))/((d - x + l*cos(theta2))*(y - l*sin(theta1) + ((y - l*sin(theta2))*(d + x - l*cos(theta1)))/(d - x + l*cos(theta2)))) - l*cos(theta2)*theta2_p - (l*cos(theta2)*(y_p - l*cos(theta2)*theta2_p))/(d - x + l*cos(theta2)) + ((l*sin(theta2)*(d + x - l*cos(theta1)) + (l*cos(theta2)*(y - l*sin(theta2))*(d + x - l*cos(theta1)))/(d - x + l*cos(theta2)))*(y_p - l*cos(theta2)*theta2_p))/((d - x + l*cos(theta2))*(y - l*sin(theta1) + ((y - l*sin(theta2))*(d + x - l*cos(theta1)))/(d - x + l*cos(theta2)))) - (l*cos(theta2)*(x_p + l*sin(theta2)*theta2_p)*(y - l*sin(theta2)))/(d - x + l*cos(theta2))^2 + ((x_p + l*sin(theta2)*theta2_p)*(l*sin(theta2)*(d + x - l*cos(theta1)) + (l*cos(theta2)*(y - l*sin(theta2))*(d + x - l*cos(theta1)))/(d - x + l*cos(theta2)))*(y - l*sin(theta2)))/((d - x + l*cos(theta2))^2*(y - l*sin(theta1) + ((y - l*sin(theta2))*(d + x - l*cos(theta1)))/(d - x + l*cos(theta2)))) - ((l*sin(theta2)*(d + x - l*cos(theta1)) + (l*cos(theta2)*(y - l*sin(theta2))*(d + x - l*cos(theta1)))/(d - x + l*cos(theta2)))*(y - l*sin(theta2))*(y_p + ((x_p + l*sin(theta1)*theta1_p)*(y - l*sin(theta2)))/(d - x + l*cos(theta2)) + ((y_p - l*cos(theta2)*theta2_p)*(d + x - l*cos(theta1)))/(d - x + l*cos(theta2)) - l*cos(theta1)*theta1_p + ((x_p + l*sin(theta2)*theta2_p)*(y - l*sin(theta2))*(d + x - l*cos(theta1)))/(d - x + l*cos(theta2))^2))/((d - x + l*cos(theta2))*(y - l*sin(theta1) + ((y - l*sin(theta2))*(d + x - l*cos(theta1)))/(d - x + l*cos(theta2)))^2) + (l*sin(theta2)*(y - l*sin(theta2))*theta2_p)/(d - x + l*cos(theta2));
 
 
J_p21 = - (l*sin(theta1)*(x_p + l*sin(theta1)*theta1_p) - l*cos(theta1)*(y_p - l*cos(theta1)*theta1_p) + l*sin(theta1)*(y - l*sin(theta1))*theta1_p + l*cos(theta1)*theta1_p*(d + x - l*cos(theta1)))/(y - l*sin(theta1) + ((y - l*sin(theta2))*(d + x - l*cos(theta1)))/(d - x + l*cos(theta2))) - ((l*cos(theta1)*(y - l*sin(theta1)) - l*sin(theta1)*(d + x - l*cos(theta1)))*(y_p + ((x_p + l*sin(theta1)*theta1_p)*(y - l*sin(theta2)))/(d - x + l*cos(theta2)) + ((y_p - l*cos(theta2)*theta2_p)*(d + x - l*cos(theta1)))/(d - x + l*cos(theta2)) - l*cos(theta1)*theta1_p + ((x_p + l*sin(theta2)*theta2_p)*(y - l*sin(theta2))*(d + x - l*cos(theta1)))/(d - x + l*cos(theta2))^2))/(y - l*sin(theta1) + ((y - l*sin(theta2))*(d + x - l*cos(theta1)))/(d - x + l*cos(theta2)))^2;
 
 
J_p22 = (l*sin(theta2)*(x_p + l*sin(theta1)*theta1_p) + l*cos(theta2)*theta2_p*(d + x - l*cos(theta1)) + (l*cos(theta2)*(x_p + l*sin(theta1)*theta1_p)*(y - l*sin(theta2)))/(d - x + l*cos(theta2)) + (l*cos(theta2)*(y_p - l*cos(theta2)*theta2_p)*(d + x - l*cos(theta1)))/(d - x + l*cos(theta2)) - (l*sin(theta2)*(y - l*sin(theta2))*theta2_p*(d + x - l*cos(theta1)))/(d - x + l*cos(theta2)) + (l*cos(theta2)*(x_p + l*sin(theta2)*theta2_p)*(y - l*sin(theta2))*(d + x - l*cos(theta1)))/(d - x + l*cos(theta2))^2)/(y - l*sin(theta1) + ((y - l*sin(theta2))*(d + x - l*cos(theta1)))/(d - x + l*cos(theta2))) - ((l*sin(theta2)*(d + x - l*cos(theta1)) + (l*cos(theta2)*(y - l*sin(theta2))*(d + x - l*cos(theta1)))/(d - x + l*cos(theta2)))*(y_p + ((x_p + l*sin(theta1)*theta1_p)*(y - l*sin(theta2)))/(d - x + l*cos(theta2)) + ((y_p - l*cos(theta2)*theta2_p)*(d + x - l*cos(theta1)))/(d - x + l*cos(theta2)) - l*cos(theta1)*theta1_p + ((x_p + l*sin(theta2)*theta2_p)*(y - l*sin(theta2))*(d + x - l*cos(theta1)))/(d - x + l*cos(theta2))^2))/(y - l*sin(theta1) + ((y - l*sin(theta2))*(d + x - l*cos(theta1)))/(d - x + l*cos(theta2)))^2;
 
% J_p = [(N11_p*D1-N11*D1_p)/D1^2, (N12_p*D1-N12*D1_p)/D1^2
%          (N21_p*D2-N21*D2_p)/D2^2, (N22_p*D2-N22*D2_p)/D2^2];

J_p = [J_p11, J_p12
    J_p21, J_p22];
     
Theta_pp = (inv(J))*[x_pp; y_pp] - J_p*[theta1_p; theta2_p];

theta1_pp = Theta_pp(1,1);
theta2_pp = Theta_pp(2,1);

== matlab function State_Flow_D/Movimento/Cinematica diretta Acc ==
  data: theta1 input; x_pp output; theta2 input; theta1_p input; theta2_p input; theta1_pp input; theta2_pp input; x input; y input; x_p input; y_p input; y_pp output
function [x_pp, y_pp] = fcn(theta1, theta2, theta1_p, theta2_p, theta1_pp, theta2_pp, x, y, x_p, y_p)

d = 0.09; 
l = 0.25;

A = x_p^2 + 2*l*sin(theta2)*x_p*theta2_p + (l*sin(theta2)*theta2_p)^2 + (x-d-l*cos(theta2))*(l*cos(theta2)*theta2_p^2 + l*sin(theta2)*theta2_pp) +...
    y_p^2 - 2*l*cos(theta2)*y_p*theta2_p + (l*cos(theta2)*theta2_p)^2 + (y-l*sin(theta2))*(l*sin(theta2)*theta2_p^2 - l*cos(theta2)*theta2_pp);

B = x_p^2 + 2*l*sin(theta1)*x_p*theta1_p + (l*sin(theta1)*theta1_p)^2 + (x+d-l*cos(theta1))*(l*cos(theta1)*theta1_p^2 + l*sin(theta1)*theta1_pp) +...
    y_p^2 - 2*l*cos(theta1)*y_p*theta1_p + (l*cos(theta1)*theta1_p)^2 + (y-l*sin(theta1))*(l*sin(theta1)*theta1_p^2 - l*cos(theta1)*theta1_pp);

y_pp = (B*(x-d-l*cos(theta2))/(x+d-l*cos(theta1)) - A)/(y-l*sin(theta2) - (x-d-l*cos(theta2))/(x+d-l*cos(theta1))*(y-l*sin(theta1)));

x_pp = (-y_pp*(y-l*sin(theta1)) - B)/(x+d-l*cos(theta1));

== matlab function State_Flow_D/Movimento/Velocita vite /Vel Asse B conv ==
  data: p input; vel_B_conv output
function vel_B_conv = fcn(p)
vel_B_conv = p  *(2*pi)/163840/64;

== matlab function State_Flow_D/Movimento/Dinamica Inversa1 ==
  data: theta1 input; C1 output; C2 output; theta2 input; theta1_p input; theta2_p input; theta1_pp input; theta2_pp input; M output; K output
function [C1, C2, M, K] = Dinamica_Inversa(theta1,theta2,theta1_p,theta2_p,theta1_pp,theta2_pp)
d = 0.09;
l = 0.25;
m = 2.9;
me = 0.36;
pv = 0.02;
Jv = 6.4e-06;
J = 5.22e-02;

A1 = cos(theta1)*theta1_p^2 + sin(theta1)*theta1_pp;
A2 = cos(theta2)*theta2_p^2 + sin(theta2)*theta2_pp;
B1 = -sin(theta1)*theta1_p^2 + cos(theta1)*theta1_pp;
B2 = -sin(theta2)*theta2_p^2 + cos(theta2)*theta2_pp;

theta3 = 2*atan((sin(theta2) - sin(theta1) + ((cos(theta2) - cos(theta1) + 18/25)^2 - ((cos(theta2) - cos(theta1) + 18/25)^2/2 +...
    (sin(theta1) - sin(theta2))^2/2)^2 + (sin(theta1) - sin(theta2))^2)^(1/2))/(cos(theta2) - cos(theta1) +...
    (cos(theta2) - cos(theta1) + 18/25)^2/2 + (sin(theta1) - sin(theta2))^2/2 + 18/25));

theta4 = -2*atan((sin(theta2) - sin(theta1) + ((cos(theta2) - cos(theta1) + 18/25)^2 - ((cos(theta2) - cos(theta1) + 18/25)^2/2 + (sin(theta1) -...
    sin(theta2))^2/2)^2 + (sin(theta1) - sin(theta2))^2)^(1/2))/(cos(theta1) - cos(theta2) + (cos(theta2) - cos(theta1) + 18/25)^2/2 +...
    (sin(theta1) -sin(theta2))^2/2 - 18/25));

N13 = cos(theta4)/sin(theta4)*sin(theta1)-cos(theta1);
N23 = cos(theta2)-cos(theta4)/sin(theta4)*sin(theta2);
D13 = cos(theta3)-cos(theta4)/sin(theta4)*sin(theta3);

theta3_p = (theta1_p*(N13)+theta2_p*(N23))/D13;

N21 = sin(theta1)*(cos(theta3)/sin(theta3) - cos(theta4)/sin(theta4)) +...
    cos(theta4)/sin(theta4)*sin(theta1) - cos(theta1);
N22 = -sin(theta2)*(cos(theta3)/sin(theta3) - cos(theta4)/sin(theta4)) -...
    cos(theta4)/sin(theta4)*sin(theta2) + cos(theta2);
D2 = sin(theta4)*(cos(theta3)/sin(theta3) - cos(theta4)/sin(theta4));

theta4_p = theta1_p*(N21/D2)+ theta2_p*(N22/D2);

J34 = [N13/D13, N23/D13; N21/D2, N22/D2];

theta3_pp = (-B1 +B2 + sin(theta3)*theta3_p^2 - sin(theta4)*theta4_p^2 + cos(theta4)/sin(theta4)*(A1 - A2 + cos(theta3)*theta3_p^2 - cos(theta4)*theta4_p^2))/...
    (cos(theta3) - cos(theta4)/sin(theta4)*sin(theta3));

theta4_pp = (A1 - A2 + cos(theta3)*theta3_p^2 - cos(theta4)*theta4_p^2 + sin(theta3)*theta3_pp)/sin(theta4);

N11 = cos(theta4)/sin(theta4)*sin(theta1)-cos(theta1);
N12 = cos(theta2)-cos(theta4)/sin(theta4)*sin(theta2);
D1 = cos(theta3)-cos(theta4)/sin(theta4)*sin(theta3);

N21 = sin(theta1)*(cos(theta3)/sin(theta3) - cos(theta4)/sin(theta4)) +...
    cos(theta4)/sin(theta4)*sin(theta1) - cos(theta1);
N22 = -sin(theta2)*(cos(theta3)/sin(theta3) - cos(theta4)/sin(theta4)) -...
    cos(theta4)/sin(theta4)*sin(theta2) + cos(theta2);
D2 = sin(theta4)*(cos(theta3)/sin(theta3) - cos(theta4)/sin(theta4));

N11p =  (-1)/(sin(theta4)^2)*theta4_p*sin(theta1) + cos(theta4)/sin(theta4)*cos(theta1)*theta1_p + sin(theta1)*theta1_p;

N12p = -(-1)/(sin(theta4)^2)*theta4_p*sin(theta2) - cos(theta4)/sin(theta4)*cos(theta2)*theta2_p - sin(theta2)*theta2_p;

D1p = -sin(theta3)*theta3_p -(-1)/(sin(theta4)^2)*theta4_p*sin(theta3) - cos(theta4)/sin(theta4)*cos(theta3)*theta3_p;

N21p = cos(theta1)*theta1_p*(cos(theta3)/sin(theta3) - cos(theta4)/sin(theta4)) + sin(theta1)*((-1)/(sin(theta3)^2)*theta3_p + 1/(sin(theta4)^2)*theta4_p) + ...
    (-1)/(sin(theta4)^2)*theta4_p*sin(theta1) + cos(theta4)/sin(theta4)*cos(theta1)*theta1_p + sin(theta1)*theta1_p;

N22p = -cos(theta2)*theta2_p*(cos(theta3)/sin(theta3) - cos(theta4)/sin(theta4)) - sin(theta2)*((-1)/(sin(theta3)^2)*theta3_p + 1/(sin(theta4)^2)*theta4_p) - ...
    (-1)/(sin(theta4)^2)*theta4_p*sin(theta2) - cos(theta4)/sin(theta4)*cos(theta2)*theta2_p - sin(theta2)*theta2_p;

D2p = cos(theta4)*theta4_p*(cos(theta3)/sin(theta3) - cos(theta4)/sin(theta4)) + sin(theta4)*((-1)/(sin(theta3)^2)*theta3_p + 1/(sin(theta4)^2)*theta4_p);

J34p = [(N11p*D1 - N11*D1p)/(D1^2), (N12p*D1 - N12*D1p)/(D1^2);(N21p*D2 - N21*D2p)/(D2^2), (N22p*D2 - N22*D2p)/(D2^2)];

J1 = [-0.5*l*sin(theta1), 0;
        0.5*l*cos(theta1), 0]; 
J1p = [-0.5*l*cos(theta1)*theta1_p, 0;
       -0.5*l*sin(theta1)*theta1_p, 0];

J2 = [0, -0.5*l*sin(theta2);
       0,  0.5*l*cos(theta2)]; 
J2p = [0, -0.5*l*cos(theta2)*theta2_p;
       0, -0.5*l*sin(theta2)*theta2_p];

J3 = [ -l*(sin(theta1)+0.5*sin(theta3)*J34(1,1)), -l*(0.5*sin(theta3)*J34(1,2));
        l*(cos(theta1)+0.5*cos(theta3)*J34(1,1)),  l*(0.5*cos(theta3)*J34(1,2))];
J3p = [ -l*(cos(theta1)*theta1_p+0.5*cos(theta3)*theta3_p*J34(1,1)+0.5*sin(theta3)*J34p(1,1)), -l*(0.5*cos(theta3)*theta3_p*J34(1,2)+0.5*sin(theta3)*J34p(1,2));
        l*(-sin(theta1)*theta1_p-0.5*sin(theta3)*theta3_p*J34(1,1)+0.5*cos(theta3)*J34p(1,1)), l*(-0.5*sin(theta3)*theta3_p*J34(1,2)+0.5*cos(theta3)*J34p(1,2))];

J4 = [ -l*0.5*sin(theta4)*J34(2,1), -l*(sin(theta2)+0.5*sin(theta4)*J34(2,2));
         l*0.5*cos(theta4)*J34(2,1),  l*(cos(theta2)+0.5*cos(theta4)*J34(2,2))];
J4p = [ -l*(0.5*cos(theta4)*theta4_p*J34(2,1)+0.5*sin(theta4)*J34p(2,1)), -l*(cos(theta2)*theta2_p+0.5*cos(theta4)*theta4_p*J34(2,2)+0.5*sin(theta4)*J34p(2,2));
        l*(-0.5*sin(theta4)*theta4_p*J34(2,1)+0.5*cos(theta4)*J34p(2,1)), l*(-sin(theta2)*theta2_p-0.5*sin(theta4)*theta4_p*J34(2,2)+0.5*cos(theta4)*J34p(2,2))];

JE = [ -l*(sin(theta1)+sin(theta3)*J34(1,1)), -l*(sin(theta3)*J34(1,2));
        l*(cos(theta1)+cos(theta3)*J34(1,1)),  l*(cos(theta3)*J34(1,2))];
JEp = [ -l*(cos(theta1)*theta1_p+cos(theta3)*theta3_p*J34(1,1)+sin(theta3)*J34p(1,1)), -l*(cos(theta3)*theta3_p*J34(1,2)+sin(theta3)*J34p(1,2));
        l*(-sin(theta1)*theta1_p-sin(theta3)*theta3_p*J34(1,1)+cos(theta3)*J34p(1,1)), l*(-sin(theta3)*theta3_p*J34(1,2)+cos(theta3)*J34p(1,2))];
  
  
M = (J*eye(2) + m*(J1')*J1 + m*(J2')*J2 + J*(J34')*J34 + m*(J3')*J3 + m*(J4')*J4 + me*(JE')*JE);
K = (m*(J1')*J1p + m*(J2')*J2p + J*(J34')*J34p + m*(J3')*J3p + m*(J4')*J4p + me*(JE')*JEp);

C = M*[theta1_pp; theta2_pp] + K*[theta1_p; theta2_p];

C1 = C(1,1);
C2 = C(2,1);

== matlab function State_Flow_D/Movimento/Velocita vite 1/Vel Asse A conv ==
  data: vA input; vel_A_conv output
function vel_A_conv = fcn(vA)
vel_A_conv = (vA)  *(2*pi)/163840/64;

== matlab function State_Flow_D/Movimento/Posizioni/Asse B conv brac1 ==
  data: p input; pos_B_conv output
function pos_B_conv = fcn(p)
pos_B_conv = p * (2*pi)/16384/64;

== matlab function State_Flow_D/Movimento/Posizioni/Asse A conv bracc ==
  data: p input; pos_B_conv output
function pos_B_conv = fcn(p)
pos_B_conv = p * (2*pi)/16384/64;

== matlab function State_Flow_D/Movimento/Velocita vite 1/Vel Asse B conv ==
  data: p input; vel_B_conv output
function vel_B_conv = fcn(p)
vel_B_conv = p  *(2*pi)/163840/64;

== matlab function State_Flow_D/Movimento/MATLAB Function2 ==
  data: x input; xp output; y input; yp output; bool input
function [xp,yp] = fcn(x, y, bool)
if bool == 4
    xp = x;
    yp = y;
else
    xp = 0;
    yp = 0;
end
